simulink model "carsim_template_v3"  (R2022b)
settings: Solver=ode3  StartTime=0.0  StopTime=10.0  FixedStep=0.001  RelTol=1e-3
settings Model: Creator=ranwe  LastModifiedBy=ranwe

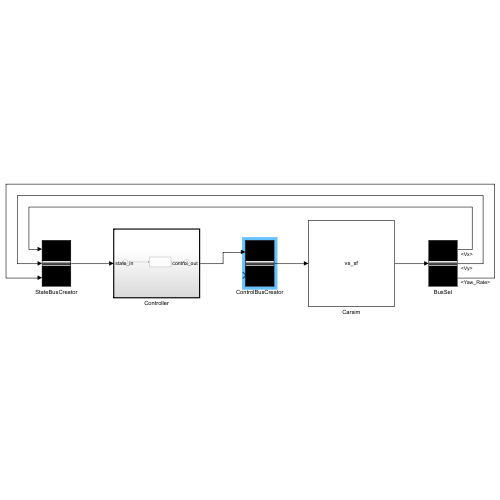
[thumbnail: Simulink's stored preview of the top-level diagram]
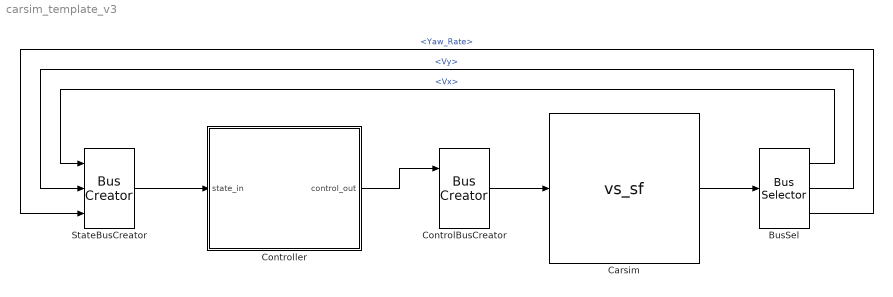
== system carsim_template_v3 ==
  BusSel : BusSelector  OutputSignals=Vx,Vy,Yaw_Rate
  Carsim : S-Function  FunctionName=vs_sf  Parameters=simfile.sim  SFunctionDeploymentMode=off  EnableBusSupport=off
  ControlBusCreator : BusCreator  Inputs=2  OutDataTypeStr=Bus: Bus_Control  NonVirtualBus=on
  Controller : Subsystem  TreatAsAtomicUnit=on
  StateBusCreator : BusCreator  Inputs=3  OutDataTypeStr=Bus: Bus_State  NonVirtualBus=on
  wires:
  Carsim/1 -> BusSel/1
  BusSel/1 -> StateBusCreator/1  "<Vx>"
  BusSel/2 -> StateBusCreator/2  "<Vy>"
  BusSel/3 -> StateBusCreator/3  "<Yaw_Rate>"
  StateBusCreator/1 -> Controller/1(state_in)
  Controller/1(control_out) -> ControlBusCreator/1
  ControlBusCreator/1 -> Carsim/1

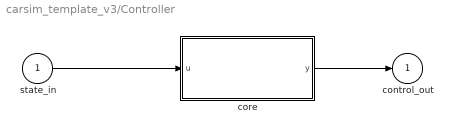
== system carsim_template_v3/Controller ==
  state_in : Inport
  core : MATLAB Function  TreatAsAtomicUnit=on
  control_out : Outport
  wires:
  state_in/1 -> core/1(u)
  core/1(y) -> control_out/1

== matlab function carsim_template_v3/Controller/core ==
  data: u input; y output
function y = fcn(u)

y = u;
